simulink library "posAug_cl"  (R2022a)
settings: Solver=VariableStepAuto  StartTime=0.0  StopTime=10.0  RelTol=1e-3
undefined symbols (not defined in the file): betaMax, elevSet, elevStart, env, FLIGHTCONTROLLER, fltCtrl, initializeBussesFromBlock, intSat, pathLaps, posAug, rollAmp, rollFreq, rollPhase, sEstim, slfAoA, slfExitTime, thetaIGain, thetaPGain, vhcl, yawAmp, yawFreq, yawPhase
libraries: slpidlib x7, simulink x3, dspsigops x3, pathFollowingCtrlAoATurb_cl x2, velocityAngle_ul x2, courseFollowLookAhead_cl x1, ctrlAllocMatrix3Comp_cl x1, eulAng2RotMat_ul x1, angleBtw2Vecs_ul x1, vrlib x1, alphaBeta_ul x1, gnd2TanRotation_ul x1
settings Model: Creator=jbfine  LastModifiedBy=jbfine

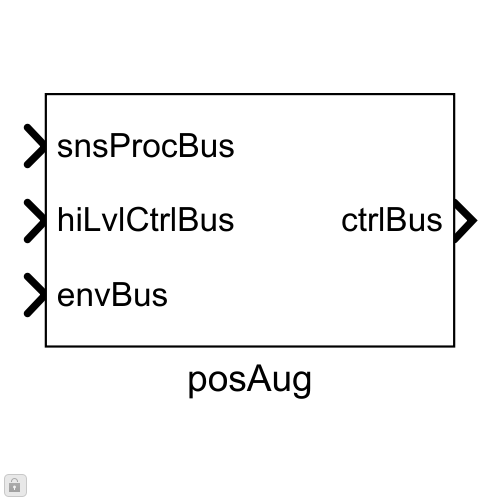
[thumbnail: Simulink's stored preview of the top-level diagram]
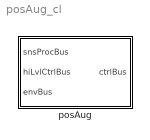
== system posAug_cl ==
  posAug : Subsystem  LoadFcn=initializeBussesFromBlock(gcb);  InitFcn=initializeBussesFromBlock(gcb);  VariantControl="strcmpi(FLIGHTCONTROLLER,\"posAug\")"  mask{initPosForInitSStar=vhcl.initPosVecGnd.Value, fluidDensity=env.water.density.Value, pathCtrl=fltCtrl, aeroStruct=vhcl.struct('OCT.aeroSurf')}
      mask prompts: initPosForInitSStar "Initial Position"; fluidDensity "Fluid Density"; pathCtrl "Controller"; aeroStruct "Aerodynamic Structure"
      settings: PreSaveFcn=initializeBussesFromBlock(gcb);
      mask DialogControl Container3 Prompt: courseFollow Params
      mask DialogControl Container4 Prompt: setpointToOutput Params

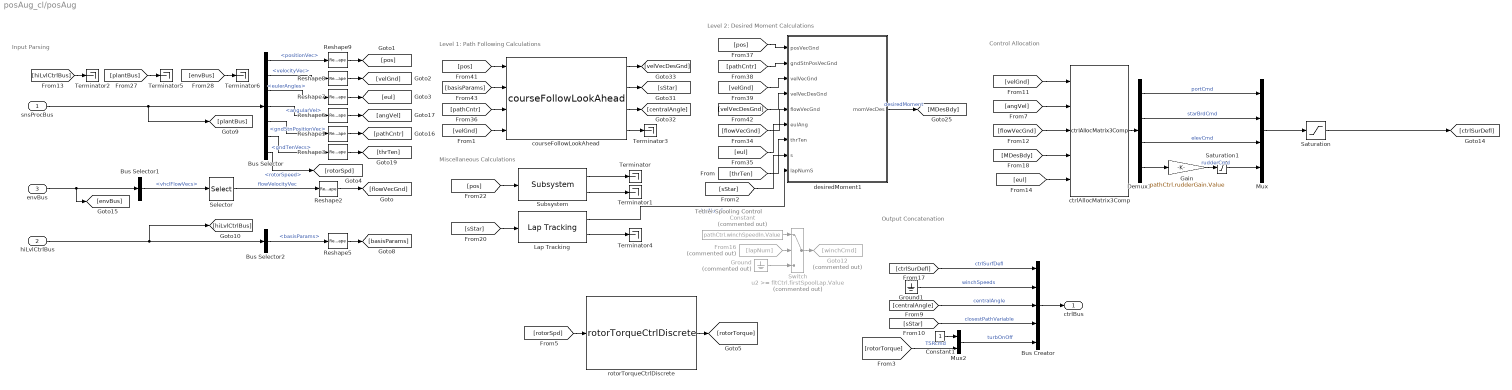
== system posAug_cl/posAug ==
  note: Level 2: Desired Moment Calculations
  note: Level 1: Path Following Calculations
  note: Input Parsing
  note: Control Allocation
  note: Tether Spooling Control
  note: Miscellaneous Calculations
  note: Output Concatenation
  snsProcBus : Inport  OutDataTypeStr=Bus: sensorsProcessingBus
  hiLvlCtrlBus : Inport  Port=2  OutDataTypeStr=Bus: hiLvlCtrlBus
  envBus : Inport  Port=3  OutDataTypeStr=Bus: envBus
  Bus Creator : BusCreator  Inputs=5
  Bus Selector : BusSelector  OutputSignals=positionVec,velocityVec,eulerAngles,angularVel,gndStnPositionVec,gndTenVecs,rotorSpeed
  Bus Selector1 : BusSelector  OutputSignals=vhclFlowVecs
  Bus Selector2 : BusSelector  OutputSignals=basisParams
  Constant : Constant  Commented=on  Value=pathCtrl.winchSpeedIn.Value
  Constant1 : Constant
  Demux1 : Demux
  From16 : From  Commented=on  GotoTag=lapNum
  Gain : Gain  Gain=pathCtrl.rudderGain.Value
  Goto12 : Goto  Commented=on  GotoTag=winchCmd
  Ground : Ground  Commented=on
  Ground1 : Ground
  Lap Tracking : pathFollowingCtrlAoATurb_cl/pathFollowingCtrlAoATurb/Lap Tracking  SystemSampleTime=-1  VariantActivationTime=update diagram  Latency=0  AutoFrameSizeCalculation=off
  Mux : Mux
  Mux2 : Mux  Inputs=2
  Reshape{1..3,5..9} (8 alike) : Reshape  OutputDimensionality=Column vector (2-D)
  Saturation : Saturate  UpperLimit=30  LowerLimit=-30
  Saturation1 : Saturate  UpperLimit=20  LowerLimit=-20
  Selector : Selector  NumberOfDimensions=2  InputPortWidth=3  IndexOptions=Select all,Index vector (dialog)  Indices=[1 3],5  OutputSizes=1,1
  Subsystem : pathFollowingCtrlAoATurb_cl/pathFollowingCtrlAoATurb/Subsystem  SystemSampleTime=-1  VariantActivationTime=update diagram  Latency=0  AutoFrameSizeCalculation=off
  Switch : Switch  Commented=on  Threshold=fltCtrl.firstSpoolLap.Value  SaturateOnIntegerOverflow=off  InputSameDT=off
  Terminator{,1..6} (7 alike) : Terminator
  courseFollowLookAhead : courseFollowLookAhead_cl/courseFollowLookAhead  SystemSampleTime=-1  VariantActivationTime=update diagram  Latency=0  AutoFrameSizeCalculation=off
  ctrlAllocMatrix3Comp : ctrlAllocMatrix3Comp_cl/ctrlAllocMatrix3Comp  aeroStruct=vhcl.struct('OCT.aeroSurf')  fluidDensity=fluidDensity  arms=vhcl.struct('OCT.thrAttch')
  desiredMoment1 : Subsystem  AncestorBlock=pathFollowingCtrlAoATurb_cl/pathFollowingCtrlAoATurb/desiredMoment1
  rotorTorqueCtrlDiscrete : rotorTorqueCtrlDiscrete/rotorTorqueCtrlDiscrete  turb_struct=vhcl.struct('OCT.turb')  rho=rho
  ctrlBus : Outport  OutDataTypeStr=Bus: fltCtrlBus  VectorParamsAs1DForOutWhenUnconnected=off
  wires:
  Lap Tracking/1 -> desiredMoment1/9(lapNumS)  "lapNumS"
  courseFollowLookAhead/1 -> [velVecDesGnd]
  [sStar] -> desiredMoment1/8(s)
  [eul] -> desiredMoment1/6(eulAng)
  Saturation/1 -> [ctrlSurDefl]
  [thrTen] -> desiredMoment1/7(thrTen)
  Demux1/3 -> Mux/3  "elevCmd"
  Bus Selector/4 -> Reshape6/1  "<angularVel>"
  [pathCntr] -> desiredMoment1/2(gndStnPosVecGnd)
  [velGnd] -> desiredMoment1/3(velVecGnd)
  Gain/1 -> Saturation1/1  "rudderCmd"
  Mux/1 -> Saturation/1
  [pathCntr] -> courseFollowLookAhead/3
  Subsystem/2 -> Terminator1/1
  [pos] -> desiredMoment1/1(posVecGnd)
  courseFollowLookAhead/4 -> Terminator3/1
  Bus Selector1/1 -> Selector/1  "<vhclFlowVecs>"
  hiLvlCtrlBus/1 -> [hiLvlCtrlBus], Bus Selector2/1
  Mux2/1 -> Bus Creator/5  "turbOnOff"
  desiredMoment1/1(momVecDes) -> [MDesBdy]  "desiredMoment"
  [hiLvlCtrlBus] -> Terminator2/1
  Ground/1 -> Switch/3
  Reshape8/1 -> [velGnd]
  Reshape6/1 -> [angVel]
  [pos] -> Subsystem/1
  Constant1/1 -> Mux2/1
  [sStar] -> Lap Tracking/1
  From16/1 -> Switch/2
  ctrlAllocMatrix3Comp/1 -> Demux1/1
  [velVecDesGnd] -> desiredMoment1/4(velVecDesGnd)
  Selector/1 -> Reshape2/1  "flowVelocityVec"
  Constant/1 -> Switch/1
  [envBus] -> Terminator6/1
  Demux1/4 -> Gain/1
  Bus Selector/5 -> Reshape1/1  "<gndStnPositionVec>"
  Bus Creator/1 -> ctrlBus/1
  [flowVecGnd] -> desiredMoment1/5(flowVecGnd)
  Reshape1/1 -> [pathCntr]
  Reshape5/1 -> [basisParams]
  Switch/1 -> Goto12/1
  [centralAngle] -> Bus Creator/3  "centralAngle"
  [MDesBdy] -> ctrlAllocMatrix3Comp/4
  [sStar] -> Bus Creator/4  "closestPathVariable"
  envBus/1 -> [envBus], Bus Selector1/1
  [eul] -> ctrlAllocMatrix3Comp/5
  Reshape9/1 -> [pos]
  [angVel] -> ctrlAllocMatrix3Comp/2
  Bus Selector/1 -> Reshape9/1  "<positionVec>"
  Reshape7/1 -> [eul]
  Demux1/1 -> Mux/1  "portCmd"
  [basisParams] -> courseFollowLookAhead/2
  [flowVecGnd] -> ctrlAllocMatrix3Comp/3
  Bus Selector/2 -> Reshape8/1  "<velocityVec>"
  Reshape2/1 -> [flowVecGnd]
  Bus Selector2/1 -> Reshape5/1  "<basisParams>"
  Lap Tracking/2 -> Terminator4/1
  Ground1/1 -> Bus Creator/2  "winchSpeeds"
  [rotorTorque] -> Mux2/2  "TSRcmd"
  Bus Selector/3 -> Reshape7/1  "<eulerAngles>"
  courseFollowLookAhead/2 -> [sStar]
  courseFollowLookAhead/3 -> [centralAngle]
  [plantBus] -> Terminator5/1
  snsProcBus/1 -> [plantBus], Bus Selector/1
  [pos] -> courseFollowLookAhead/1
  Demux1/2 -> Mux/2  "starBrdCmd"
  Reshape3/1 -> [thrTen]
  Bus Selector/6 -> Reshape3/1  "<gndTenVecs>"
  [ctrlSurDefl] -> Bus Creator/1  "ctrlSurfDefl"
  Subsystem/1 -> Terminator/1
  [velGnd] -> courseFollowLookAhead/4
  [velGnd] -> ctrlAllocMatrix3Comp/1
  rotorTorqueCtrlDiscrete/1 -> [rotorTorque]
  [rotorSpd] -> rotorTorqueCtrlDiscrete/1
  Bus Selector/7 -> [rotorSpd]  "<rotorSpeed>"
  Saturation1/1 -> Mux/4

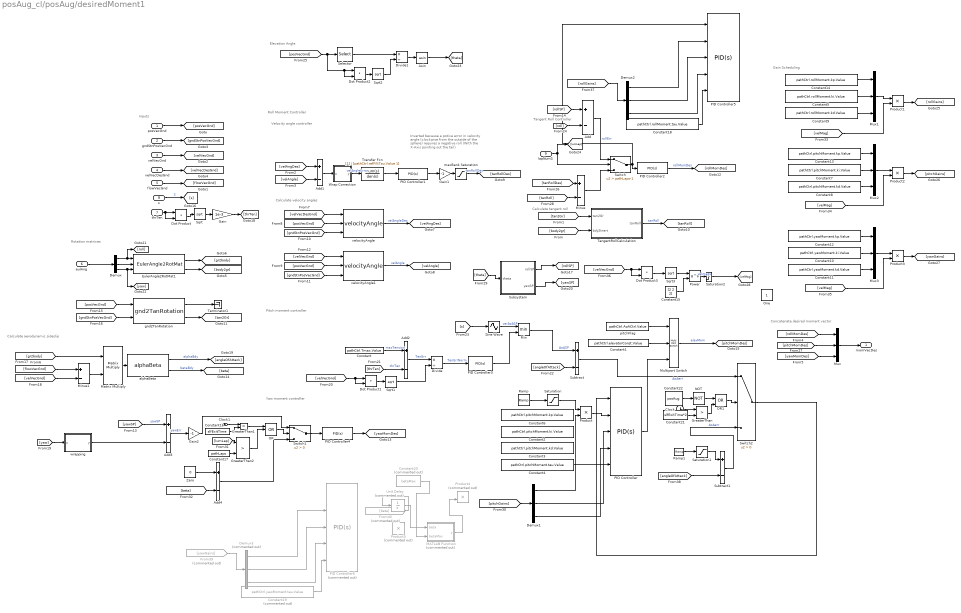
== system posAug_cl/posAug/desiredMoment1 ==
  note: Elevation Angle
  note: Yaw moment controller
  note: Pitch moment controller
  note: Inverted because a potive error
      | in velocity angle (clockwise from the
      | outside of the sphere) requires a negative
      | roll (With the X-Axis pointing out the tail)
  note: Velocity angle controller
  note: Inputs
  note: Rotation matrices
  note: Calculate velocity angles
  note: Calculate tangent roll
  note: Tangent Roll Controller
  note: Concatenate desired moment vector
  note: Calculate aerodynamic sideslip
  note: Roll Moment Controller
  note: Gain Scheduling
  posVecGnd : Inport
  gndStnPosVecGnd : Inport  Port=2
  velVecGnd : Inport  Port=3
  velVecDesGnd : Inport  Port=4
  flowVecGnd : Inport  Port=5
  eulAng : Inport  Port=6
  thrTen : Inport  Port=7
  s : Inport  Port=8
  lapNumS : Inport  Port=9
  Add{,1..4} (5 alike) : Sum  Inputs=+-
  Asin : Trigonometry  Operator=asin
  Clock : Clock
  Clock1 : Clock
  Constant : Constant  Value=pathCtrl.Tmax.Value
  Constant1 : Constant  Value=pathCtrl.elevatorConst.Value
  Constant10 : Constant  Value=pathCtrl.yawMoment.ki.Value
  Constant11 : Constant  Value=pathCtrl.yawMoment.kd.Value
  Constant12 : Constant  Value=pathCtrl.yawMoment.kp.Value
  Constant13 : Constant  Value=pathCtrl.pitchMoment.kp.Value
  Constant14 : Constant  Value=pathCtrl.rollMoment.kp.Value
  Constant15 : Constant  Value=[2 2 2]
  Constant16 : Constant  Value=slfExitTime
  Constant17 : Constant  Value=pathLaps
  Constant18 : Constant  Value=pathCtrl.rollMoment.tau.Value
  Constant19 : Constant  Commented=on  Value=pathCtrl.yawMoment.tau.Value
  Constant2 : Constant  Value=pathCtrl.pitchMoment.ki.Value
  Constant20 : Constant  Commented=on  Value=betaMax
  Constant21 : Constant  Value=slfExitTime*2
  Constant22 : Constant  Value=posAug
  Constant3 : Constant  Value=pathCtrl.pitchMoment.kd.Value
  Constant4 : Constant  Value=pathCtrl.pitchMoment.tau.Value
  Constant5 : Constant  Value=pathCtrl.rollMoment.ki.Value
  Constant6 : Constant  Value=pathCtrl.pitchMoment.kp.Value
  Constant7 : Constant  Value=pathCtrl.pitchMoment.ki.Value
  Constant8 : Constant  Value=pathCtrl.pitchMoment.kd.Value
  Constant9 : Constant  Value=pathCtrl.rollMoment.kd.Value
  Demux : Demux  Outputs=3
  Demux1 : Demux  Outputs=3
  Demux2 : Demux  Outputs=3
  Demux3 : Demux  Commented=on  Outputs=3
  Divide : Product  Inputs=*/
  Divide1 : Product  Inputs=*/
  Dot Product{,1..3} (4 alike) : DotProduct  OutDataTypeStr=Inherit: Inherit via internal rule
  EulerAngle2RotMat1 : eulAng2RotMat_ul/EulerAngle2RotMat  SystemSampleTime=-1  VariantActivationTime=update diagram  Latency=0  AutoFrameSizeCalculation=off
  From39 : From  Commented=on  GotoTag=yawGains
  From40 : From  Commented=on  GotoTag=beta
  Gain : Gain  Gain=1e-3
  Gain1 : Gain  Gain=-1
  Gain2 : Gain  Gain=-1
  GreaterThan : RelationalOperator  Operator=>  OutDataTypeStr=boolean  RndMeth=Simplest  InputSameDT=off
  GreaterThan1 : RelationalOperator  Operator=>  OutDataTypeStr=boolean  RndMeth=Simplest  InputSameDT=off
  GreaterThan2 : RelationalOperator  Operator=>  OutDataTypeStr=boolean  RndMeth=Simplest  InputSameDT=off
  MATLAB Function : MATLAB Function  Commented=on  TreatAsAtomicUnit=on
  Matrix Multiply : Product  Multiplication=Matrix(*)
  Min : MinMax  Inputs=2
  Minus : Sum  Inputs=+-
  Minus1 : Sum  Inputs=+-
  Multiport Switch : MultiPortSwitch  DataPortOrder=Specify indices  Inputs=2  DataPortIndices={0,1}  SaturateOnIntegerOverflow=off  InputSameDT=off
  Mux{,1..3} (4 alike) : Mux  Inputs=3
  NOT : Logic  Operator=NOT  IconShape=distinctive  AllPortsSameDT=off  OutDataTypeStr=boolean
  OR : Logic  Operator=OR  Inputs=3  IconShape=distinctive  AllPortsSameDT=off  OutDataTypeStr=boolean
  OR1 : Logic  Operator=OR  IconShape=distinctive  AllPortsSameDT=off  OutDataTypeStr=boolean
  One : Constant  OutDataTypeStr=Inherit: Inherit via back propagation
  PID Controller : slpidlib/PID Controller  Controller=PID  Form=Parallel  TimeDomain=Continuous-time  UseExternalTs=off  SampleTime=-1  IntegratorMethod=Forward Euler  FilterMethod=Forward Euler  ControllerParametersSource=external  P=pathCtrl.pitchMoment.kp.Value  I=pathCtrl.pitchMoment.ki.Value  UseKiTs=off  D=pathCtrl.pitchMoment.kd.Value  N=1/pathCtrl.pitchMoment.tau.Value  UseFilter=on  TunerSelectOption=Transfer Function Based (PID Tuner App)  InitialConditionSource=internal  InitialConditionForIntegrator=0  InitialConditionForFilter=0  DifferentiatorICPrevScaledInput=0  ExternalReset=none  TrackingMode=off  Kt=1  LimitOutput=off  SatLimitsSource=internal  UpperSaturationLimit=inf  LowerSaturationLimit=-100  LinearizeAsGain=on  AntiWindupMode=clamping  Kb=1  POutMin=[]  POutMax=[]  IOutMin=[]  IOutMax=[]  DOutMin=[]  DOutMax=[]  NOutMin=[]  NOutMax=[]  SumOutMin=[]  SumOutMax=[]  SaturationOutMin=[]  SaturationOutMax=[]  PParamMin=[]  PParamMax=[]  IParamMin=[]  IParamMax=[]  DParamMin=[]  DParamMax=[]  NParamMin=[]  NParamMax=[]  KbParamMin=[]  KbParamMax=[]  KtParamMin=[]  KtParamMax=[]  KbOutMin=[]  KbOutMax=[]  KtOutMin=[]  KtOutMax=[]  IntegratorOutMin=[]  IntegratorOutMax=[]  FilterOutMin=[]  FilterOutMax=[]  SumI1OutMin=[]  SumI1OutMax=[]  SumI2OutMin=[]  SumI2OutMax=[]  SumI3OutMin=[]  SumI3OutMax=[]  SumI4OutMin=[]  SumI4OutMax=[]  SumDOutMin=[]  SumDOutMax=[]  DifferentiatorOutMin=[]  DifferentiatorOutMax=[]  FilterDiffOutCoefMin=[]  FilterDiffOutCoefMax=[]  ReciprocalOutMin=[]  ReciprocalOutMax=[]  SumDenOutMin=[]  SumDenOutMax=[]  SumNumOutMin=[]  SumNumOutMax=[]  DivideOutMin=[]  DivideOutMax=[]  UdiffTsProdOutMin=[]  UdiffTsProdOutMax=[]  NTsProdOutMin=[]  NTsProdOutMax=[]  UintegralTsProdOutMin=[]  UintegralTsProdOutMax=[]  UngainTsProdOutMin=[]  UngainTsProdOutMax=[]  IntegratorContinuousStateAttributes=''  IntegratorStateMustResolveToSignalObject=off  IntegratorRTWStateStorageClass=Auto  FilterContinuousStateAttributes=''  FilterStateMustResolveToSignalObject=off  FilterRTWStateStorageClass=Auto  ParallelPVariant=ExternalParameters  IdealPVariant=Disabled  IVariant=ExternalParameters  DVariant=ExternalParameters  IntegratorVariant=Continuous  SatVariant=Disabled  AWVariant=Passthrough  PCopyVariant=Disabled  TRVariant=Disabled  FdbkBlocksVariant=Forward  IdealPFdbkVariant=Disabled  SatFdbkVariant=Disabled  DerivativeFilterVariant=ContFilter  NVariant=ExternalParameters  NCopyVariant=Disabled  FilterICVariant=InternalICsFilter  IntegratorICVariant=InternalICs  ExternalResetVariant=Disabled  TRSumVariant=Passthrough  SumFdbkVariant=Disabled  SumVariant=Sum_PID  TsampFilterVariant=InternalTs  TsampNgainVariant=Passthrough  TsampIntegralVariant=Passthrough  ExternalSaturationOutDataTypeStr=Inherit: Same as second input  aMode=0
  PID Controller1 : slpidlib/PID Controller  Controller=PID  Form=Parallel  TimeDomain=Continuous-time  UseExternalTs=off  SampleTime=-1  IntegratorMethod=Forward Euler  FilterMethod=Forward Euler  ControllerParametersSource=internal  P=pathCtrl.tanRoll.kp.Value  I=pathCtrl.tanRoll.ki.Value  UseKiTs=off  D=pathCtrl.tanRoll.kd.Value  N=1/pathCtrl.tanRoll.tau.Value  UseFilter=on  TunerSelectOption=Transfer Function Based (PID Tuner App)  InitialConditionSource=internal  InitialConditionForIntegrator=0  InitialConditionForFilter=0  DifferentiatorICPrevScaledInput=0  ExternalReset=none  TrackingMode=off  Kt=1  LimitOutput=off  SatLimitsSource=internal  UpperSaturationLimit=inf  LowerSaturationLimit=-100  LinearizeAsGain=on  AntiWindupMode=clamping  Kb=1  POutMin=[]  POutMax=[]  IOutMin=[]  IOutMax=[]  DOutMin=[]  DOutMax=[]  NOutMin=[]  NOutMax=[]  SumOutMin=[]  SumOutMax=[]  SaturationOutMin=[]  SaturationOutMax=[]  PParamMin=[]  PParamMax=[]  IParamMin=[]  IParamMax=[]  DParamMin=[]  DParamMax=[]  NParamMin=[]  NParamMax=[]  KbParamMin=[]  KbParamMax=[]  KtParamMin=[]  KtParamMax=[]  KbOutMin=[]  KbOutMax=[]  KtOutMin=[]  KtOutMax=[]  IntegratorOutMin=[]  IntegratorOutMax=[]  FilterOutMin=[]  FilterOutMax=[]  SumI1OutMin=[]  SumI1OutMax=[]  SumI2OutMin=[]  SumI2OutMax=[]  SumI3OutMin=[]  SumI3OutMax=[]  SumI4OutMin=[]  SumI4OutMax=[]  SumDOutMin=[]  SumDOutMax=[]  DifferentiatorOutMin=[]  DifferentiatorOutMax=[]  FilterDiffOutCoefMin=[]  FilterDiffOutCoefMax=[]  ReciprocalOutMin=[]  ReciprocalOutMax=[]  SumDenOutMin=[]  SumDenOutMax=[]  SumNumOutMin=[]  SumNumOutMax=[]  DivideOutMin=[]  DivideOutMax=[]  UdiffTsProdOutMin=[]  UdiffTsProdOutMax=[]  NTsProdOutMin=[]  NTsProdOutMax=[]  UintegralTsProdOutMin=[]  UintegralTsProdOutMax=[]  UngainTsProdOutMin=[]  UngainTsProdOutMax=[]  IntegratorContinuousStateAttributes=''  IntegratorStateMustResolveToSignalObject=off  IntegratorRTWStateStorageClass=Auto  FilterContinuousStateAttributes=''  FilterStateMustResolveToSignalObject=off  FilterRTWStateStorageClass=Auto  ParallelPVariant=InternalParameters  IdealPVariant=Disabled  IVariant=InternalParameters  DVariant=InternalParameters  IntegratorVariant=Continuous  SatVariant=Disabled  AWVariant=Passthrough  PCopyVariant=Disabled  TRVariant=Disabled  FdbkBlocksVariant=Forward  IdealPFdbkVariant=Disabled  SatFdbkVariant=Disabled  DerivativeFilterVariant=ContFilter  NVariant=InternalParameters  NCopyVariant=Disabled  FilterICVariant=InternalICsFilter  IntegratorICVariant=InternalICs  ExternalResetVariant=Disabled  TRSumVariant=Passthrough  SumFdbkVariant=Disabled  SumVariant=Sum_PID  TsampFilterVariant=InternalTs  TsampNgainVariant=Passthrough  TsampIntegralVariant=Passthrough  ExternalSaturationOutDataTypeStr=Inherit: Same as second input  aMode=0
  PID Controller2 : slpidlib/PID Controller  Controller=PID  Form=Parallel  TimeDomain=Continuous-time  UseExternalTs=off  SampleTime=-1  IntegratorMethod=Forward Euler  FilterMethod=Forward Euler  ControllerParametersSource=internal  P=pathCtrl.rollMoment.kp.Value  I=pathCtrl.rollMoment.ki.Value  UseKiTs=off  D=pathCtrl.rollMoment.kd.Value  N=1/pathCtrl.rollMoment.tau.Value  UseFilter=on  TunerSelectOption=Transfer Function Based (PID Tuner App)  InitialConditionSource=internal  InitialConditionForIntegrator=0  InitialConditionForFilter=0  DifferentiatorICPrevScaledInput=0  ExternalReset=none  TrackingMode=off  Kt=1  LimitOutput=off  SatLimitsSource=internal  UpperSaturationLimit=inf  LowerSaturationLimit=-100  LinearizeAsGain=on  AntiWindupMode=clamping  Kb=1  POutMin=[]  POutMax=[]  IOutMin=[]  IOutMax=[]  DOutMin=[]  DOutMax=[]  NOutMin=[]  NOutMax=[]  SumOutMin=[]  SumOutMax=[]  SaturationOutMin=[]  SaturationOutMax=[]  PParamMin=[]  PParamMax=[]  IParamMin=[]  IParamMax=[]  DParamMin=[]  DParamMax=[]  NParamMin=[]  NParamMax=[]  KbParamMin=[]  KbParamMax=[]  KtParamMin=[]  KtParamMax=[]  KbOutMin=[]  KbOutMax=[]  KtOutMin=[]  KtOutMax=[]  IntegratorOutMin=[]  IntegratorOutMax=[]  FilterOutMin=[]  FilterOutMax=[]  SumI1OutMin=[]  SumI1OutMax=[]  SumI2OutMin=[]  SumI2OutMax=[]  SumI3OutMin=[]  SumI3OutMax=[]  SumI4OutMin=[]  SumI4OutMax=[]  SumDOutMin=[]  SumDOutMax=[]  DifferentiatorOutMin=[]  DifferentiatorOutMax=[]  FilterDiffOutCoefMin=[]  FilterDiffOutCoefMax=[]  ReciprocalOutMin=[]  ReciprocalOutMax=[]  SumDenOutMin=[]  SumDenOutMax=[]  SumNumOutMin=[]  SumNumOutMax=[]  DivideOutMin=[]  DivideOutMax=[]  UdiffTsProdOutMin=[]  UdiffTsProdOutMax=[]  NTsProdOutMin=[]  NTsProdOutMax=[]  UintegralTsProdOutMin=[]  UintegralTsProdOutMax=[]  UngainTsProdOutMin=[]  UngainTsProdOutMax=[]  IntegratorContinuousStateAttributes=''  IntegratorStateMustResolveToSignalObject=off  IntegratorRTWStateStorageClass=Auto  FilterContinuousStateAttributes=''  FilterStateMustResolveToSignalObject=off  FilterRTWStateStorageClass=Auto  ParallelPVariant=InternalParameters  IdealPVariant=Disabled  IVariant=InternalParameters  DVariant=InternalParameters  IntegratorVariant=Continuous  SatVariant=Disabled  AWVariant=Passthrough  PCopyVariant=Disabled  TRVariant=Disabled  FdbkBlocksVariant=Forward  IdealPFdbkVariant=Disabled  SatFdbkVariant=Disabled  DerivativeFilterVariant=ContFilter  NVariant=InternalParameters  NCopyVariant=Disabled  FilterICVariant=InternalICsFilter  IntegratorICVariant=InternalICs  ExternalResetVariant=Disabled  TRSumVariant=Passthrough  SumFdbkVariant=Disabled  SumVariant=Sum_PID  TsampFilterVariant=InternalTs  TsampNgainVariant=Passthrough  TsampIntegralVariant=Passthrough  ExternalSaturationOutDataTypeStr=Inherit: Same as second input  aMode=0
  PID Controller3 : slpidlib/PID Controller  Controller=PID  Form=Parallel  TimeDomain=Continuous-time  UseExternalTs=off  SampleTime=-1  IntegratorMethod=Forward Euler  FilterMethod=Forward Euler  ControllerParametersSource=internal  P=pathCtrl.alphaCtrl.kp.Value  I=pathCtrl.alphaCtrl.ki.Value  UseKiTs=off  D=pathCtrl.alphaCtrl.kd.Value  N=1/pathCtrl.alphaCtrl.tau.Value  UseFilter=on  TunerSelectOption=Transfer Function Based (PID Tuner App)  InitialConditionSource=internal  InitialConditionForIntegrator=0  InitialConditionForFilter=0  DifferentiatorICPrevScaledInput=0  ExternalReset=none  TrackingMode=off  Kt=1  LimitOutput=on  SatLimitsSource=internal  UpperSaturationLimit=pathCtrl.AoAConst.Value  LowerSaturationLimit=pathCtrl.AoAmin.Value  LinearizeAsGain=on  AntiWindupMode=clamping  Kb=1  POutMin=[]  POutMax=[]  IOutMin=[]  IOutMax=[]  DOutMin=[]  DOutMax=[]  NOutMin=[]  NOutMax=[]  SumOutMin=[]  SumOutMax=[]  SaturationOutMin=[]  SaturationOutMax=[]  PParamMin=[]  PParamMax=[]  IParamMin=[]  IParamMax=[]  DParamMin=[]  DParamMax=[]  NParamMin=[]  NParamMax=[]  KbParamMin=[]  KbParamMax=[]  KtParamMin=[]  KtParamMax=[]  KbOutMin=[]  KbOutMax=[]  KtOutMin=[]  KtOutMax=[]  IntegratorOutMin=[]  IntegratorOutMax=[]  FilterOutMin=[]  FilterOutMax=[]  SumI1OutMin=[]  SumI1OutMax=[]  SumI2OutMin=[]  SumI2OutMax=[]  SumI3OutMin=[]  SumI3OutMax=[]  SumI4OutMin=[]  SumI4OutMax=[]  SumDOutMin=[]  SumDOutMax=[]  DifferentiatorOutMin=[]  DifferentiatorOutMax=[]  FilterDiffOutCoefMin=[]  FilterDiffOutCoefMax=[]  ReciprocalOutMin=[]  ReciprocalOutMax=[]  SumDenOutMin=[]  SumDenOutMax=[]  SumNumOutMin=[]  SumNumOutMax=[]  DivideOutMin=[]  DivideOutMax=[]  UdiffTsProdOutMin=[]  UdiffTsProdOutMax=[]  NTsProdOutMin=[]  NTsProdOutMax=[]  UintegralTsProdOutMin=[]  UintegralTsProdOutMax=[]  UngainTsProdOutMin=[]  UngainTsProdOutMax=[]  IntegratorContinuousStateAttributes=''  IntegratorStateMustResolveToSignalObject=off  IntegratorRTWStateStorageClass=Auto  FilterContinuousStateAttributes=''  FilterStateMustResolveToSignalObject=off  FilterRTWStateStorageClass=Auto  ParallelPVariant=InternalParameters  IdealPVariant=Disabled  IVariant=InternalParameters  DVariant=InternalParameters  IntegratorVariant=Continuous  SatVariant=Enabled  AWVariant=ContClampingParallel  PCopyVariant=Disabled  TRVariant=Disabled  FdbkBlocksVariant=Forward  IdealPFdbkVariant=Disabled  SatFdbkVariant=Disabled  DerivativeFilterVariant=ContFilter  NVariant=InternalParameters  NCopyVariant=Disabled  FilterICVariant=InternalICsFilter  IntegratorICVariant=InternalICs  ExternalResetVariant=Disabled  TRSumVariant=Passthrough  SumFdbkVariant=Disabled  SumVariant=Sum_PID  TsampFilterVariant=InternalTs  TsampNgainVariant=Passthrough  TsampIntegralVariant=Passthrough  ExternalSaturationOutDataTypeStr=Inherit: Same as second input  aMode=0
  PID Controller4 : slpidlib/PID Controller  Controller=PID  Form=Parallel  TimeDomain=Continuous-time  UseExternalTs=off  SampleTime=-1  IntegratorMethod=Forward Euler  FilterMethod=Forward Euler  ControllerParametersSource=internal  P=pathCtrl.yawMoment.kp.Value  I=pathCtrl.yawMoment.ki.Value  UseKiTs=off  D=pathCtrl.yawMoment.kd.Value  N=1/pathCtrl.yawMoment.tau.Value  UseFilter=on  TunerSelectOption=Transfer Function Based (PID Tuner App)  InitialConditionSource=internal  InitialConditionForIntegrator=0  InitialConditionForFilter=0  DifferentiatorICPrevScaledInput=0  ExternalReset=none  TrackingMode=off  Kt=1  LimitOutput=off  SatLimitsSource=internal  UpperSaturationLimit=inf  LowerSaturationLimit=-100  LinearizeAsGain=on  AntiWindupMode=clamping  Kb=1  POutMin=[]  POutMax=[]  IOutMin=[]  IOutMax=[]  DOutMin=[]  DOutMax=[]  NOutMin=[]  NOutMax=[]  SumOutMin=[]  SumOutMax=[]  SaturationOutMin=[]  SaturationOutMax=[]  PParamMin=[]  PParamMax=[]  IParamMin=[]  IParamMax=[]  DParamMin=[]  DParamMax=[]  NParamMin=[]  NParamMax=[]  KbParamMin=[]  KbParamMax=[]  KtParamMin=[]  KtParamMax=[]  KbOutMin=[]  KbOutMax=[]  KtOutMin=[]  KtOutMax=[]  IntegratorOutMin=[]  IntegratorOutMax=[]  FilterOutMin=[]  FilterOutMax=[]  SumI1OutMin=[]  SumI1OutMax=[]  SumI2OutMin=[]  SumI2OutMax=[]  SumI3OutMin=[]  SumI3OutMax=[]  SumI4OutMin=[]  SumI4OutMax=[]  SumDOutMin=[]  SumDOutMax=[]  DifferentiatorOutMin=[]  DifferentiatorOutMax=[]  FilterDiffOutCoefMin=[]  FilterDiffOutCoefMax=[]  ReciprocalOutMin=[]  ReciprocalOutMax=[]  SumDenOutMin=[]  SumDenOutMax=[]  SumNumOutMin=[]  SumNumOutMax=[]  DivideOutMin=[]  DivideOutMax=[]  UdiffTsProdOutMin=[]  UdiffTsProdOutMax=[]  NTsProdOutMin=[]  NTsProdOutMax=[]  UintegralTsProdOutMin=[]  UintegralTsProdOutMax=[]  UngainTsProdOutMin=[]  UngainTsProdOutMax=[]  IntegratorContinuousStateAttributes=''  IntegratorStateMustResolveToSignalObject=off  IntegratorRTWStateStorageClass=Auto  FilterContinuousStateAttributes=''  FilterStateMustResolveToSignalObject=off  FilterRTWStateStorageClass=Auto  ParallelPVariant=InternalParameters  IdealPVariant=Disabled  IVariant=InternalParameters  DVariant=InternalParameters  IntegratorVariant=Continuous  SatVariant=Disabled  AWVariant=Passthrough  PCopyVariant=Disabled  TRVariant=Disabled  FdbkBlocksVariant=Forward  IdealPFdbkVariant=Disabled  SatFdbkVariant=Disabled  DerivativeFilterVariant=ContFilter  NVariant=InternalParameters  NCopyVariant=Disabled  FilterICVariant=InternalICsFilter  IntegratorICVariant=InternalICs  ExternalResetVariant=Disabled  TRSumVariant=Passthrough  SumFdbkVariant=Disabled  SumVariant=Sum_PID  TsampFilterVariant=InternalTs  TsampNgainVariant=Passthrough  TsampIntegralVariant=Passthrough  ExternalSaturationOutDataTypeStr=Inherit: Same as second input  aMode=0
  PID Controller5 : slpidlib/PID Controller  Controller=PID  Form=Parallel  TimeDomain=Continuous-time  UseExternalTs=off  SampleTime=-1  IntegratorMethod=Forward Euler  FilterMethod=Forward Euler  ControllerParametersSource=external  P=pathCtrl.pitchMoment.kp.Value  I=pathCtrl.pitchMoment.ki.Value  UseKiTs=off  D=pathCtrl.pitchMoment.kd.Value  N=1/pathCtrl.pitchMoment.tau.Value  UseFilter=on  TunerSelectOption=Transfer Function Based (PID Tuner App)  InitialConditionSource=internal  InitialConditionForIntegrator=0  InitialConditionForFilter=0  DifferentiatorICPrevScaledInput=0  ExternalReset=none  TrackingMode=off  Kt=1  LimitOutput=off  SatLimitsSource=internal  UpperSaturationLimit=inf  LowerSaturationLimit=-100  LinearizeAsGain=on  AntiWindupMode=clamping  Kb=1  POutMin=[]  POutMax=[]  IOutMin=[]  IOutMax=[]  DOutMin=[]  DOutMax=[]  NOutMin=[]  NOutMax=[]  SumOutMin=[]  SumOutMax=[]  SaturationOutMin=[]  SaturationOutMax=[]  PParamMin=[]  PParamMax=[]  IParamMin=[]  IParamMax=[]  DParamMin=[]  DParamMax=[]  NParamMin=[]  NParamMax=[]  KbParamMin=[]  KbParamMax=[]  KtParamMin=[]  KtParamMax=[]  KbOutMin=[]  KbOutMax=[]  KtOutMin=[]  KtOutMax=[]  IntegratorOutMin=[]  IntegratorOutMax=[]  FilterOutMin=[]  FilterOutMax=[]  SumI1OutMin=[]  SumI1OutMax=[]  SumI2OutMin=[]  SumI2OutMax=[]  SumI3OutMin=[]  SumI3OutMax=[]  SumI4OutMin=[]  SumI4OutMax=[]  SumDOutMin=[]  SumDOutMax=[]  DifferentiatorOutMin=[]  DifferentiatorOutMax=[]  FilterDiffOutCoefMin=[]  FilterDiffOutCoefMax=[]  ReciprocalOutMin=[]  ReciprocalOutMax=[]  SumDenOutMin=[]  SumDenOutMax=[]  SumNumOutMin=[]  SumNumOutMax=[]  DivideOutMin=[]  DivideOutMax=[]  UdiffTsProdOutMin=[]  UdiffTsProdOutMax=[]  NTsProdOutMin=[]  NTsProdOutMax=[]  UintegralTsProdOutMin=[]  UintegralTsProdOutMax=[]  UngainTsProdOutMin=[]  UngainTsProdOutMax=[]  IntegratorContinuousStateAttributes=''  IntegratorStateMustResolveToSignalObject=off  IntegratorRTWStateStorageClass=Auto  FilterContinuousStateAttributes=''  FilterStateMustResolveToSignalObject=off  FilterRTWStateStorageClass=Auto  ParallelPVariant=ExternalParameters  IdealPVariant=Disabled  IVariant=ExternalParameters  DVariant=ExternalParameters  IntegratorVariant=Continuous  SatVariant=Disabled  AWVariant=Passthrough  PCopyVariant=Disabled  TRVariant=Disabled  FdbkBlocksVariant=Forward  IdealPFdbkVariant=Disabled  SatFdbkVariant=Disabled  DerivativeFilterVariant=ContFilter  NVariant=ExternalParameters  NCopyVariant=Disabled  FilterICVariant=InternalICsFilter  IntegratorICVariant=InternalICs  ExternalResetVariant=Disabled  TRSumVariant=Passthrough  SumFdbkVariant=Disabled  SumVariant=Sum_PID  TsampFilterVariant=InternalTs  TsampNgainVariant=Passthrough  TsampIntegralVariant=Passthrough  ExternalSaturationOutDataTypeStr=Inherit: Same as second input  aMode=0
  PID Controller6 : slpidlib/PID Controller  Commented=on  Controller=PID  Form=Parallel  TimeDomain=Continuous-time  UseExternalTs=off  SampleTime=-1  IntegratorMethod=Forward Euler  FilterMethod=Forward Euler  ControllerParametersSource=external  P=pathCtrl.pitchMoment.kp.Value  I=pathCtrl.pitchMoment.ki.Value  UseKiTs=off  D=pathCtrl.pitchMoment.kd.Value  N=1/pathCtrl.pitchMoment.tau.Value  UseFilter=on  TunerSelectOption=Transfer Function Based (PID Tuner App)  InitialConditionSource=internal  InitialConditionForIntegrator=0  InitialConditionForFilter=0  DifferentiatorICPrevScaledInput=0  ExternalReset=none  TrackingMode=off  Kt=1  LimitOutput=off  SatLimitsSource=internal  UpperSaturationLimit=inf  LowerSaturationLimit=-100  LinearizeAsGain=on  AntiWindupMode=clamping  Kb=1  POutMin=[]  POutMax=[]  IOutMin=[]  IOutMax=[]  DOutMin=[]  DOutMax=[]  NOutMin=[]  NOutMax=[]  SumOutMin=[]  SumOutMax=[]  SaturationOutMin=[]  SaturationOutMax=[]  PParamMin=[]  PParamMax=[]  IParamMin=[]  IParamMax=[]  DParamMin=[]  DParamMax=[]  NParamMin=[]  NParamMax=[]  KbParamMin=[]  KbParamMax=[]  KtParamMin=[]  KtParamMax=[]  KbOutMin=[]  KbOutMax=[]  KtOutMin=[]  KtOutMax=[]  IntegratorOutMin=[]  IntegratorOutMax=[]  FilterOutMin=[]  FilterOutMax=[]  SumI1OutMin=[]  SumI1OutMax=[]  SumI2OutMin=[]  SumI2OutMax=[]  SumI3OutMin=[]  SumI3OutMax=[]  SumI4OutMin=[]  SumI4OutMax=[]  SumDOutMin=[]  SumDOutMax=[]  DifferentiatorOutMin=[]  DifferentiatorOutMax=[]  FilterDiffOutCoefMin=[]  FilterDiffOutCoefMax=[]  ReciprocalOutMin=[]  ReciprocalOutMax=[]  SumDenOutMin=[]  SumDenOutMax=[]  SumNumOutMin=[]  SumNumOutMax=[]  DivideOutMin=[]  DivideOutMax=[]  UdiffTsProdOutMin=[]  UdiffTsProdOutMax=[]  NTsProdOutMin=[]  NTsProdOutMax=[]  UintegralTsProdOutMin=[]  UintegralTsProdOutMax=[]  UngainTsProdOutMin=[]  UngainTsProdOutMax=[]  IntegratorContinuousStateAttributes=''  IntegratorStateMustResolveToSignalObject=off  IntegratorRTWStateStorageClass=Auto  FilterContinuousStateAttributes=''  FilterStateMustResolveToSignalObject=off  FilterRTWStateStorageClass=Auto  ParallelPVariant=ExternalParameters  IdealPVariant=Disabled  IVariant=ExternalParameters  DVariant=ExternalParameters  IntegratorVariant=Continuous  SatVariant=Disabled  AWVariant=Passthrough  PCopyVariant=Disabled  TRVariant=Disabled  FdbkBlocksVariant=Forward  IdealPFdbkVariant=Disabled  SatFdbkVariant=Disabled  DerivativeFilterVariant=ContFilter  NVariant=ExternalParameters  NCopyVariant=Disabled  FilterICVariant=InternalICsFilter  IntegratorICVariant=InternalICs  ExternalResetVariant=Disabled  TRSumVariant=Passthrough  SumFdbkVariant=Disabled  SumVariant=Sum_PID  TsampFilterVariant=InternalTs  TsampNgainVariant=Passthrough  TsampIntegralVariant=Passthrough  ExternalSaturationOutDataTypeStr=Inherit: Same as second input  aMode=0
  Power : Math  Operator=pow
  Product{,1..3} (4 alike) : Product
  Product4 : Product  Commented=on
  Product5 : Product  Commented=on
  Ramp : simulink/Sources/Ramp  slope=0.05  start=100  InitialOutput=0.2
  Ramp1 : simulink/Sources/Ramp  slope=0.005  start=slfExitTime  InitialOutput=slfAoA
  Saturation : Saturate  UpperLimit=1  LowerLimit=0.2
  Saturation1 : Saturate  UpperLimit=7.5*pi/180  LowerLimit=slfAoA
  Saturation2 : Saturate  UpperLimit=1000  LowerLimit=1
  Selector : Selector  InputPortWidth=3  IndexOptions=Index vector (dialog)  Indices=[3]  OutputSizes=1
  Sine Wave : Sin  TimeSource=Use external signal  Amplitude=0  Bias=fltCtrl.AoAConst.Value  Frequency=4*pi  Phase=pi/2  SampleTime=0
  Sqrt{,1..3} (4 alike) : Sqrt
  Subsystem : Subsystem
  Subtract : Sum  Inputs=+-
  Subtract1 : Sum  Inputs=+-
  Switch : Switch  Criteria=u2 > Threshold  Threshold=pathLaps-1  SaturateOnIntegerOverflow=off  InputSameDT=off
  Switch1 : Switch  Criteria=u2 > Threshold  SaturateOnIntegerOverflow=off  InputSameDT=off
  Switch2 : Switch  Criteria=u2 > Threshold  SaturateOnIntegerOverflow=off  InputSameDT=off
  TangentRollCalculation : Subsystem
  Terminator1 : Terminator
  Transfer Fcn : TransferFcn  Denominator=[pathCtrl.refFiltTau.Value 1]
  Unit Delay : UnitDelay  Commented=on  SampleTime=-1  HasFrameUpgradeWarning=on
  Wrap Correction : Subsystem
  Zero : Constant  Value=0  OutDataTypeStr=Inherit: Inherit via back propagation
  alphaBeta : alphaBeta_ul/alphaBeta  SystemSampleTime=-1  VariantActivationTime=update diagram  Latency=0  AutoFrameSizeCalculation=off
  gnd2TanRotation : gnd2TanRotation_ul/gnd2TanRotation  SystemSampleTime=-1  VariantActivationTime=update diagram  Latency=0  AutoFrameSizeCalculation=off
  maxBank Saturation : Saturate  UpperLimit=pathCtrl.maxBank.upperLimit.Value  LowerLimit=pathCtrl.maxBank.lowerLimit.Value
  pitchFlag : Constant  Value=pathCtrl.AoACtrl.Value
  velocityAngle : velocityAngle_ul/velocityAngle  SystemSampleTime=-1  VariantActivationTime=update diagram  Latency=0  AutoFrameSizeCalculation=off
  velocityAngle1 : velocityAngle_ul/velocityAngle  SystemSampleTime=-1  VariantActivationTime=update diagram  Latency=0  AutoFrameSizeCalculation=off
  wrapping : MATLAB Function  TreatAsAtomicUnit=on
  momVecDes : Outport  VectorParamsAs1DForOutWhenUnconnected=off
  wires:
  Min/1 -> Subtract/1  "AoASP"
  PID Controller3/1 -> Min/2
  Sine Wave/1 -> Min/1  "varAoASP"
  [s] -> Sine Wave/1
  s/1 -> [s]  "S"
  Saturation/1 -> Product/1
  Product/1 -> PID Controller/2
  Ramp/1 -> Saturation/1
  Constant4/1 -> PID Controller/5
  Divide/1 -> PID Controller3/1  "TenErrNorm"
  Constant/1 -> Add2/1  "maxTension"
  Sqrt1/1 -> Divide/2
  Add2/1 -> Divide/1  "TenErr"
  [thrTen] -> Add2/2  "thrTen"
  Transfer Fcn/1 -> PID Controller1/1
  Mux/1 -> momVecDes/1
  Demux/3 -> [yaw], EulerAngle2RotMat1/3
  Dot Product1/1 -> Sqrt1/1
  [velVecGnd] -> Dot Product1/1, Dot Product1/2
  Gain/1 -> [thrTen]
  Dot Product/1 -> Sqrt/1
  Sqrt/1 -> Gain/1
  thrTen/1 -> Dot Product/1, Dot Product/2
  PID Controller/1 -> Multiport Switch/3
  Constant1/1 -> Multiport Switch/2
  [angleOfAttack] -> Subtract/2
  pitchFlag/1 -> Multiport Switch/1
  Multiport Switch/1 -> [pitchMomDes]  "elevMom"
  [pitchMomDes] -> Mux/2
  PID Controller1/1 -> Gain1/1
  [yawMomDes] -> Mux/3
  gnd2TanRotation/1 -> Terminator1/1
  gnd2TanRotation/2 -> [tan2Gr]
  [gndStnPosVecGnd] -> gnd2TanRotation/2
  [posVecGnd] -> gnd2TanRotation/1
  [rollSP] -> Add/1
  [roll] -> Add/2
  [velVecGnd] -> velocityAngle1/1
  [gndStnPosVecGnd] -> velocityAngle1/3
  [gndStnPosVecGnd] -> velocityAngle/3
  [posVecGnd] -> velocityAngle1/2
  [posVecGnd] -> velocityAngle/2
  [velVecDesGnd] -> velocityAngle/1
  [velAngle] -> Add1/2
  [velAngDes] -> Add1/1
  velocityAngle1/1 -> [velAngle]  "velAngle"
  velocityAngle/1 -> [velAngDes]  "velAngleDes"
  velVecDesGnd/1 -> [velVecDesGnd]
  gndStnPosVecGnd/1 -> [gndStnPosVecGnd]
  alphaBeta/1 -> [angleOfAttack]  "alphaBdy"
  alphaBeta/2 -> [beta]  "betaBdy"
  Matrix Multiply/1 -> alphaBeta/1
  [gr2body] -> Matrix Multiply/1
  [body2gr] -> TangentRollCalculation/2(bdy2Inert)
  EulerAngle2RotMat1/1 -> [gr2body]
  EulerAngle2RotMat1/2 -> [body2gr]
  Demux/2 -> EulerAngle2RotMat1/2
  eulAng/1 -> Demux/1
  [flowVecGnd] -> Minus1/1
  [velVecGnd] -> Minus1/2
  Minus1/1 -> Matrix Multiply/2
  TangentRollCalculation/1(tanRoll) -> [tanRoll]  "tanRoll"
  [tan2Gr] -> TangentRollCalculation/1(tan2Gr)
  flowVecGnd/1 -> [flowVecGnd]
  Add1/1 -> Wrap Correction/1(u)
  maxBank Saturation/1 -> [tanRollDes]  "tanRollDes"
  Gain1/1 -> maxBank Saturation/1
  Add/1 -> Switch/1  "rollErr"
  velVecGnd/1 -> [velVecGnd]
  posVecGnd/1 -> [posVecGnd]
  Wrap Correction/1(y) -> Transfer Fcn/1  "velAngleError"
  [rollMomDes] -> Mux/1
  Subsystem/1(rollSP) -> [rollSP]
  Subsystem/2(yawSP) -> [yawSP]
  [yawSP] -> Add3/1  "yawSP"
  Demux/1 -> [roll], EulerAngle2RotMat1/1
  [yaw] -> wrapping/1(u)
  Switch/1 -> PID Controller2/1, PID Controller5/1
  Minus/1 -> Switch/3
  [tanRollDes] -> Minus/1
  [tanRoll] -> Minus/2
  [posVecGnd] -> Dot Product2/2, Dot Product2/1, Selector/1
  Dot Product2/1 -> Sqrt2/1
  Selector/1 -> Divide1/1
  Sqrt2/1 -> Divide1/2
  Divide1/1 -> Asin/1
  Asin/1 -> [theta]
  [theta] -> Subsystem/1(theta)
  lapNumS/1 -> Switch/2, [lumLap]
  [lumLap] -> GreaterThan2/1
  [beta] -> Add4/2
  Zero/1 -> Add4/1
  Add3/1 -> Gain2/1  "yawErr"
  Constant11/1 -> Mux3/3
  Product3/1 -> [yawGains]
  Product2/1 -> [pitchGains]
  Mux3/1 -> Product3/1
  Product1/1 -> [rollGains]
  Constant7/1 -> Mux2/2
  Constant14/1 -> Mux1/1
  Mux2/1 -> Product2/1
  [velMag] -> Product1/2
  Constant9/1 -> Mux1/3
  Constant8/1 -> Mux2/3
  Mux1/1 -> Product1/1
  Constant13/1 -> Mux2/1
  Constant12/1 -> Mux3/1
  Constant10/1 -> Mux3/2
  Constant5/1 -> Mux1/2
  [velMag] -> Product2/2
  [velMag] -> Product3/2
  [velVecGnd] -> Dot Product3/1, Dot Product3/2
  Sqrt3/1 -> Power/1
  Constant15/1 -> Power/2
  Dot Product3/1 -> Sqrt3/1
  Clock/1 -> GreaterThan/1
  [angleOfAttack] -> Subtract1/2
  Ramp1/1 -> Saturation1/1
  Saturation1/1 -> Subtract1/1
  Clock1/1 -> GreaterThan1/1
  wrapping/1(y) -> Add3/2
  Gain2/1 -> Switch1/1
  Subtract/1 -> Switch2/1  "AoAerr"
  GreaterThan1/1 -> OR/1
  OR/1 -> Switch1/2
  Constant16/1 -> GreaterThan1/2
  Constant17/1 -> GreaterThan2/2
  GreaterThan2/1 -> OR/2
  [pitchGains] -> Demux1/1
  Demux1/1 -> Product/2
  Demux1/2 -> PID Controller/3
  Demux1/3 -> PID Controller/4
  Power/1 -> Saturation2/1  "velmags"
  Saturation2/1 -> [velMag]
  PID Controller4/1 -> [yawMomDes]
  Switch1/1 -> PID Controller4/1
  Add4/1 -> Switch1/3
  Demux2/2 -> PID Controller5/3
  Demux2/1 -> PID Controller5/2
  Constant18/1 -> PID Controller5/5
  [rollGains] -> Demux2/1
  Demux2/3 -> PID Controller5/4
  From39/1 -> Demux3/1
  Constant19/1 -> PID Controller6/5
  Demux3/1 -> PID Controller6/2
  Demux3/2 -> PID Controller6/3
  Demux3/3 -> PID Controller6/4
  PID Controller2/1 -> [rollMomDes]  "rollMomDes"
  From40/1 -> Unit Delay/1
  Constant20/1 -> MATLAB Function/2(betaMax)
  Unit Delay/1 -> MATLAB Function/1(beta)
  MATLAB Function/1(y) -> Product4/2
  Subtract1/1 -> Switch2/3  "AoAerr"
  Switch2/1 -> PID Controller/1
  Constant21/1 -> GreaterThan/2
  OR1/1 -> Switch2/2
  GreaterThan/1 -> OR1/2
  NOT/1 -> OR1/1
  Constant22/1 -> NOT/1

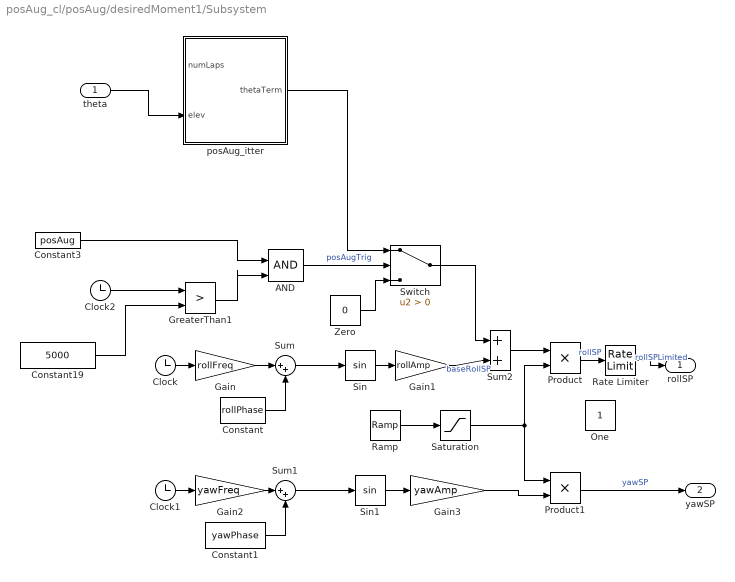
== system posAug_cl/posAug/desiredMoment1/Subsystem ==
  theta : Inport
  AND : Logic  IconShape=distinctive  AllPortsSameDT=off  OutDataTypeStr=boolean
  Clock : Clock
  Clock1 : Clock
  Clock2 : Clock
  Constant : Constant  Value=rollPhase
  Constant1 : Constant  Value=yawPhase
  Constant19 : Constant  Value=5000
  Constant3 : Constant  Value=posAug
  Gain : Gain  Gain=rollFreq
  Gain1 : Gain  Gain=rollAmp
  Gain2 : Gain  Gain=yawFreq
  Gain3 : Gain  Gain=yawAmp
  GreaterThan1 : RelationalOperator  Operator=>  OutDataTypeStr=boolean  RndMeth=Simplest  InputSameDT=off
  One : Constant  OutDataTypeStr=Inherit: Inherit via back propagation
  Product : Product
  Product1 : Product
  Ramp : simulink/Sources/Ramp  slope=1/(8*pi/rollFreq)  start=slfExitTime  InitialOutput=0
  Rate Limiter : RateLimiter  SampleTimeMode=inherited
  Saturation : Saturate  UpperLimit=1  LowerLimit=0
  Sin : Trigonometry
  Sin1 : Trigonometry
  Sum : Sum  Inputs=|++
  Sum1 : Sum  Inputs=|++
  Sum2 : Sum  Inputs=|++
  Switch : Switch  Criteria=u2 > Threshold  SaturateOnIntegerOverflow=off  InputSameDT=off
  Zero : Constant  Value=0  OutDataTypeStr=Inherit: Inherit via back propagation
  posAug_itter : Subsystem
  rollSP : Outport
  yawSP : Outport  Port=2
  wires:
  Clock/1 -> Gain/1
  Gain/1 -> Sum/1
  Sum/1 -> Sin/1
  Constant/1 -> Sum/2
  Sin/1 -> Gain1/1
  Gain1/1 -> Sum2/2  "baseRollSP"
  theta/1 -> posAug_itter/2(elev)
  Gain3/1 -> Product1/2
  Clock1/1 -> Gain2/1
  Sum1/1 -> Sin1/1
  Constant1/1 -> Sum1/2
  Gain2/1 -> Sum1/1
  Sin1/1 -> Gain3/1
  Rate Limiter/1 -> rollSP/1  "rollSPLimited"
  Product1/1 -> yawSP/1  "yawSP"
  Ramp/1 -> Saturation/1
  Sum2/1 -> Product/1
  posAug_itter/1(thetaTerm) -> Switch/1
  Zero/1 -> Switch/3
  Switch/1 -> Sum2/1
  Product/1 -> Rate Limiter/1  "rollSP"
  Constant19/1 -> GreaterThan1/2
  GreaterThan1/1 -> AND/2
  Constant3/1 -> AND/1
  AND/1 -> Switch/2  "posAugTrig"
  Saturation/1 -> Product/2, Product1/1
  Clock2/1 -> GreaterThan1/1

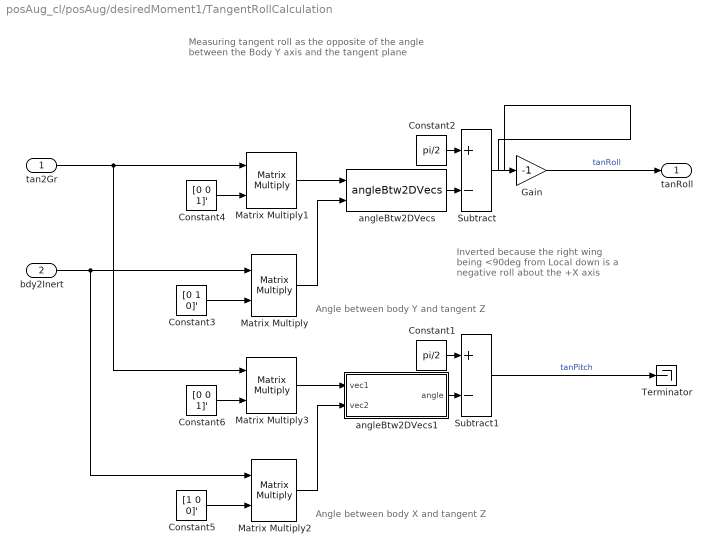
== system posAug_cl/posAug/desiredMoment1/TangentRollCalculation ==
  note: Angle between body X and tangent Z
  note: Inverted because the right wing
      | being <90deg from Local down
      | is a negative roll about the +X axis
  note: Angle between body Y and tangent Z
  note: Measuring tangent roll as the opposite
      | of the angle between the Body Y axis
      | and the tangent plane
  tan2Gr : Inport
  bdy2Inert : Inport  Port=2
  Constant1 : Constant  Value=pi/2
  Constant2 : Constant  Value=pi/2
  Constant3 : Constant  Value=[0 1 0]'
  Constant4 : Constant  Value=[0 0 1]'
  Constant5 : Constant  Value=[1 0 0]'
  Constant6 : Constant  Value=[0 0 1]'
  Gain : Gain  Gain=-1
  Matrix Multiply{,1..3} (4 alike) : Product  Multiplication=Matrix(*)
  Subtract : Sum  Inputs=+-
  Subtract1 : Sum  Inputs=+-
  Terminator : Terminator
  angleBtw2DVecs : angleBtw2Vecs_ul/angleBtw2DVecs  SystemSampleTime=-1  VariantActivationTime=update diagram  Latency=0  AutoFrameSizeCalculation=off
  angleBtw2DVecs1 : Subsystem
  tanRoll : Outport  VectorParamsAs1DForOutWhenUnconnected=off
  wires:
  Constant5/1 -> Matrix Multiply2/2
  angleBtw2DVecs1/1(angle) -> Subtract1/2
  Constant1/1 -> Subtract1/1
  Matrix Multiply3/1 -> angleBtw2DVecs1/1(vec1)
  Constant6/1 -> Matrix Multiply3/2
  Matrix Multiply2/1 -> angleBtw2DVecs1/2(vec2)
  tan2Gr/1 -> Matrix Multiply1/1, Matrix Multiply3/1
  Subtract1/1 -> Terminator/1  "tanPitch"
  bdy2Inert/1 -> Matrix Multiply/1, Matrix Multiply2/1
  Gain/1 -> tanRoll/1  "tanRoll"
  Matrix Multiply/1 -> angleBtw2DVecs/2
  Constant4/1 -> Matrix Multiply1/2
  Matrix Multiply1/1 -> angleBtw2DVecs/1
  Constant2/1 -> Subtract/1
  angleBtw2DVecs/1 -> Subtract/2
  Constant3/1 -> Matrix Multiply/2
  Subtract/1 -> Gain/1

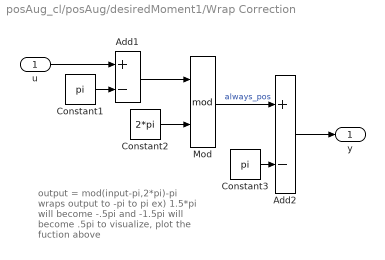
== system posAug_cl/posAug/desiredMoment1/Wrap Correction ==
  note: output = mod(input-pi,2*pi)-pi
      | wraps output to -pi to pi
      |
      | ex) 1.5*pi will become -.5pi
      | 	and -1.5pi will become .5pi
      |
      | to visualize, plot the fuction above
  u : Inport
  Add1 : Sum  Inputs=+-
  Add2 : Sum  Inputs=+-
  Constant1 : Constant  Value=pi
  Constant2 : Constant  Value=2*pi
  Constant3 : Constant  Value=pi
  Mod : Math  Operator=mod  SignedPower=on
  y : Outport  VectorParamsAs1DForOutWhenUnconnected=off
  wires:
  Add2/1 -> y/1
  Constant3/1 -> Add2/2
  Mod/1 -> Add2/1  "always_pos"
  Constant2/1 -> Mod/2
  Add1/1 -> Mod/1
  Constant1/1 -> Add1/2
  u/1 -> Add1/1

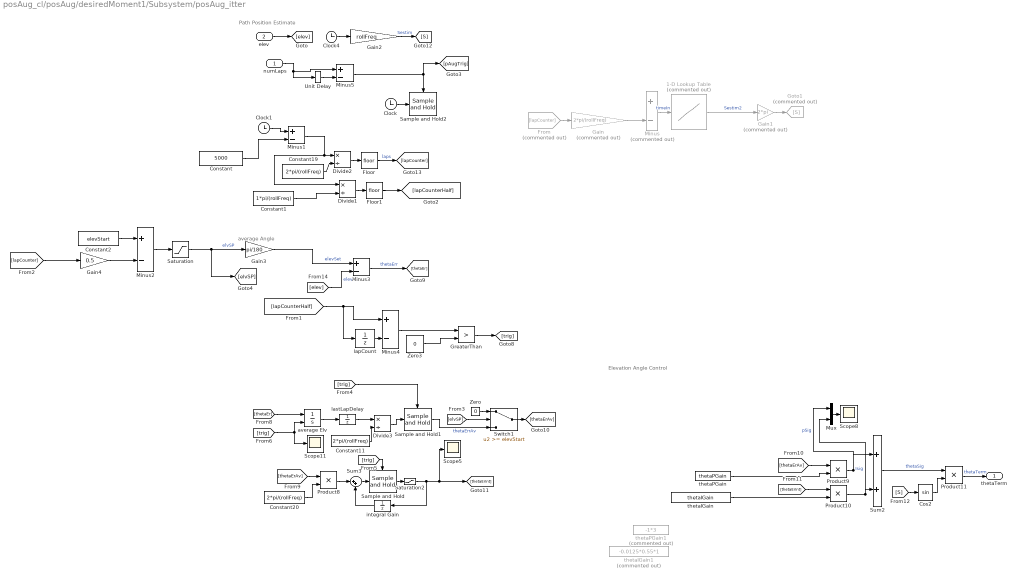
== system posAug_cl/posAug/desiredMoment1/Subsystem/posAug_itter ==
  note: average Angle
  note: Path Position Estimate
  note: Elevation Angle Control
  numLaps : Inport
  elev : Inport  Port=2
  1-D Lookup Table : Lookup_n-D  Commented=on  NumberOfTableDimensions=1  BreakpointsForDimension1=times  Table=sEstim  ExtrapMethod=Clip  InternalRulePriority=Speed  RndMeth=Simplest
  Clock : Clock
  Clock1 : Clock
  Clock4 : Clock
  Constant : Constant  Value=5000
  Constant1 : Constant  Value=1*pi/(rollFreq)
  Constant11 : Constant  Value=2*pi/(rollFreq)
  Constant19 : Constant  Value=2*pi/(rollFreq)
  Constant2 : Constant  Value=elevStart
  Constant20 : Constant  Value=2*pi/(rollFreq)
  Cos2 : Trigonometry
  Divide1 : Product  Inputs=*/
  Divide2 : Product  Inputs=*/
  Divide3 : Product  Inputs=*/
  Floor : Rounding
  Floor1 : Rounding
  From : From  Commented=on  GotoTag=lapCounter
  Gain : Gain  Commented=on  Gain=2*pi/(rollFreq)
  Gain1 : Gain  Commented=on  Gain=2*pi
  Gain2 : Gain  Gain=rollFreq
  Gain3 : Gain  Gain=pi/180
  Gain4 : Gain  Gain=0.5
  Goto1 : Goto  Commented=on  GotoTag=S
  GreaterThan : RelationalOperator  Operator=>  OutDataTypeStr=boolean  RndMeth=Simplest  InputSameDT=off
  Minus : Sum  Commented=on  Inputs=+-
  Minus{1..5} (5 alike) : Sum  Inputs=+-
  Mux : Mux  Inputs=2
  Product{8..11} (4 alike) : Product
  Sample and Hold : dspsigops/Sample and Hold  trig=Rising edge  initCond=0  latchinput=off
  Sample and Hold1 : dspsigops/Sample and Hold  trig=Rising edge  initCond=0  latchinput=off
  Sample and Hold2 : dspsigops/Sample and Hold  trig=Rising edge  initCond=0  latchinput=off
  Saturation : Saturate  UpperLimit=elevStart  LowerLimit=elevSet
  Saturation2 : Saturate  UpperLimit=intSat  LowerLimit=-intSat
  Scope11 : Scope
  Scope5 : Scope
  Scope8 : Scope
  Sum2 : Sum  Inputs=|++
  Sum3 : Sum  Inputs=|++
  Switch1 : Switch  Threshold=elevStart  SaturateOnIntegerOverflow=off  InputSameDT=off
  Unit Delay : UnitDelay  SampleTime=-1  HasFrameUpgradeWarning=on
  Zero : Constant  Value=0  OutDataTypeStr=Inherit: Inherit via back propagation
  Zero3 : Constant  Value=0  OutDataTypeStr=Inherit: Inherit via back propagation
  average Elv : Integrator  ExternalReset=rising
  integral Gain : UnitDelay  SampleTime=-1  HasFrameUpgradeWarning=on
  lapCount : UnitDelay  SampleTime=-1  HasFrameUpgradeWarning=on
  lastLapDelay : UnitDelay  SampleTime=-1  HasFrameUpgradeWarning=on
  thetaIGain : Constant  Value=thetaIGain
  thetaIGain1 : Constant  Commented=on  Value=-0.0125*0.55*1
  thetaPGain : Constant  Value=thetaPGain
  thetaPGain1 : Constant  Commented=on  Value=-1*3
  thetaTerm : Outport
  wires:
  Sum2/1 -> Product11/1  "thetaSig"
  [thetaErAv] -> Product8/1
  lapCount/1 -> Minus4/2
  thetaIGain/1 -> Product10/2
  Product11/1 -> thetaTerm/1  "thetaTerm"
  GreaterThan/1 -> [trig]
  thetaPGain/1 -> Product9/2
  [trig] -> Scope11/1, average Elv/2
  [thetaErInt] -> Product10/1
  [elev] -> Minus3/2  "elev"
  average Elv/1 -> lastLapDelay/1
  Divide2/1 -> Floor/1
  Zero3/1 -> GreaterThan/2
  Floor/1 -> [lapCounter]  "laps"
  Product10/1 -> Mux/2, Sum2/2  "Isig"
  Mux/1 -> Scope8/1
  Product9/1 -> Mux/1, Sum2/1  "pSig"
  Cos2/1 -> Product11/2
  Saturation2/1 -> Scope5/1, [thetaErInt], integral Gain/1
  Sample and Hold1/1 -> Switch1/3  "thetaErrAv"
  Product8/1 -> Sum3/1
  [S] -> Cos2/1
  [trig] -> Sample and Hold1/Trigger
  [thetaErAv] -> Product9/1
  Constant20/1 -> Product8/2
  Sample and Hold/1 -> Saturation2/1
  integral Gain/1 -> Sum3/2
  Minus1/1 -> Divide1/1, Divide2/1
  Divide3/1 -> Sample and Hold1/1
  Clock4/1 -> Gain2/1
  Saturation/1 -> [elvSP], Gain3/1  "elvSP"
  Constant11/1 -> Divide3/2
  Gain2/1 -> [S]  "Sestim"
  [trig] -> Sample and Hold/Trigger
  lastLapDelay/1 -> Divide3/1
  Minus3/1 -> [thetaEr]  "thetaErr"
  Minus4/1 -> GreaterThan/1
  [thetaEr] -> average Elv/1
  Sum3/1 -> Sample and Hold/1
  Constant19/1 -> Divide2/2
  Clock1/1 -> Minus1/1
  elev/1 -> [elev]
  Minus5/1 -> [pAugTrig], Sample and Hold2/Trigger
  Clock/1 -> Sample and Hold2/1
  From/1 -> Gain/1
  Gain/1 -> Minus/2
  Minus/1 -> 1-D Lookup Table/1  "timeIn"
  1-D Lookup Table/1 -> Gain1/1  "Sestim2"
  Gain1/1 -> Goto1/1
  Divide1/1 -> Floor1/1
  Floor1/1 -> [lapCounterHalf]
  Constant1/1 -> Divide1/2
  [lapCounter] -> Gain4/1
  Constant2/1 -> Minus2/1
  Minus2/1 -> Saturation/1
  Gain3/1 -> Minus3/1  "elevSet"
  numLaps/1 -> Unit Delay/1, Minus5/1
  Unit Delay/1 -> Minus5/2
  [elvSP] -> Switch1/2
  Zero/1 -> Switch1/1
  Switch1/1 -> [thetaErAv]
  Gain4/1 -> Minus2/2
  Constant/1 -> Minus1/2
  [lapCounterHalf] -> lapCount/1, Minus4/1

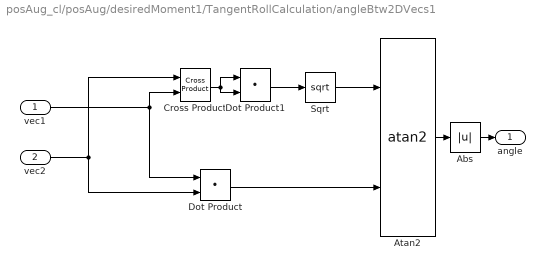
== system posAug_cl/posAug/desiredMoment1/TangentRollCalculation/angleBtw2DVecs1 ==
  vec1 : Inport
  vec2 : Inport  Port=2
  Abs : Abs  SaturateOnIntegerOverflow=off
  Atan2 : Trigonometry  Operator=atan2
  Cross Product : vrlib/Utilities/Cross Product
  Dot Product : DotProduct  OutDataTypeStr=Inherit: Inherit via internal rule
  Dot Product1 : DotProduct  OutDataTypeStr=Inherit: Inherit via internal rule
  Sqrt : Sqrt
  angle : Outport  VectorParamsAs1DForOutWhenUnconnected=off
  wires:
  Sqrt/1 -> Atan2/1
  Dot Product1/1 -> Sqrt/1
  Abs/1 -> angle/1
  Dot Product/1 -> Atan2/2
  Cross Product/1 -> Dot Product1/2, Dot Product1/1
  vec2/1 -> Dot Product/2, Cross Product/1
  vec1/1 -> Cross Product/2, Dot Product/1
  Atan2/1 -> Abs/1

== matlab function posAug_cl/posAug/desiredMoment1/wrapping ==
  data: u input; y output
function y = fcn(u)

if abs(u)>2*pi
y=rem(u,2*pi);
else
    y=u;
end

== matlab function posAug_cl/posAug/desiredMoment1/MATLAB Function ==
  data: beta input; y output; betaMax input
function y = fcn(beta, betaMax)

if abs(beta)>betaMax

y=1-((abs(beta)-betaMax)/(betaMax));
else
    y=1;
end
end
